simulink model "HPGR"  (Simulink 7.5)
settings: Solver=ode45  StartTime=0.0  StopTime=100  RelTol=1e-3
settings Model: Creator=Lucho  LastModifiedBy=Lucho

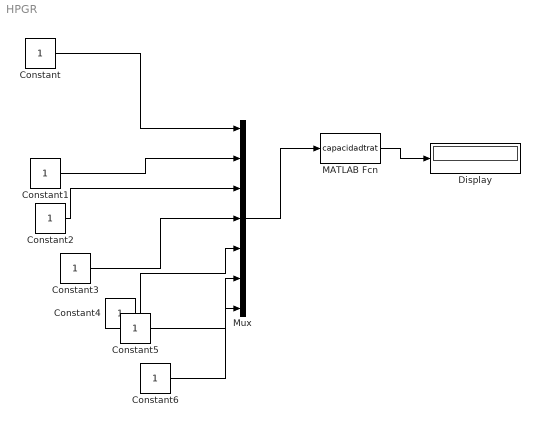
== system HPGR ==
  Constant{,1..6} (7 alike) : Constant  OutDataType=fixdt(1, 16)  OutScaling=2^0
  Display : Display
  MATLAB Fcn : MATLABFcn  MATLABFcn=capacidadtrat
  Mux : Mux  Inputs=7
  wires:
  Constant/1 -> Mux/1
  Constant1/1 -> Mux/2
  Constant2/1 -> Mux/3
  Constant3/1 -> Mux/4
  Constant4/1 -> Mux/5
  Constant5/1 -> Mux/6
  Constant6/1 -> Mux/7
  Mux/1 -> MATLAB Fcn/1
  MATLAB Fcn/1 -> Display/1
